simulink model "Cw2"  (R2016b)
settings: Solver=VariableStepDiscrete  StartTime=0.0  StopTime=2e-3  RelTol=1e-3
libraries: dspsrcs4 x4, dsparch4 x2, commutil2 x2, commchan3 x1, commseqgen3 x1
settings Model: Creator=Krzysztof  LastModifiedBy=Krzysztof

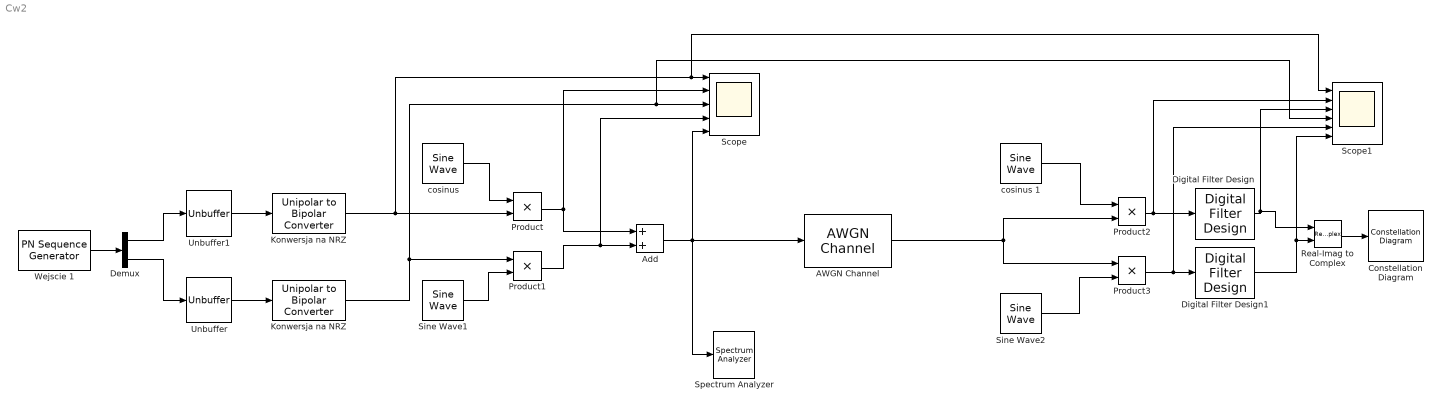
== system Cw2 ==
  AWGN Channel : commchan3/AWGN Channel  InputProcessing=Columns as channels (frame based)  seed=67  noiseMode="Signal to noise ratio  (Eb/No)"  EbNodB=20  EsNodB=10  SNRdB=30  bitsPerSym=2  Ps=1  Tsym=1/500e3  variance=1
  Add : Sum
  Constellation Diagram : ConstellationDiagram
  Demux : Demux  Outputs=2
  Digital Filter Design : dsparch4/Digital Filter Design  mwdsp_browser_bugfix_var=off
  Digital Filter Design1 : dsparch4/Digital Filter Design  mwdsp_browser_bugfix_var=off
  Konwersja na NRZ : commutil2/Unipolar to Bipolar Converter  M=2  polarity=Positive  dataType=Inherit via internal rule
  "Konwersja na NRZ " : commutil2/Unipolar to Bipolar Converter  M=2  polarity=Positive  dataType=Inherit via internal rule
  Product{,1..3} (4 alike) : Product
  Real-Imag to Complex : RealImagToComplex  SampleTime=1/400e6
  Scope : Scope  NumInputPorts=5
  Scope1 : Scope  NumInputPorts=6
  Sine Wave1 : dspsrcs4/Sine Wave  Amplitude=-1  Frequency=40e6  Phase=0  SampleMode=Discrete  OutComplex=Real  CompMethod=Trigonometric fcn  TableSize=Speed  SampleTime=1/400e6  SamplesPerFrame=1  ResetState=Restart at time zero  OutputFrames=off  dataType=double  wordLen=16  udDataType=sfix(16)  fracBitsMode=Best precision  numFracBits=15  OutDataTypeStr=double  LastOutDataTypeStr=double
  Sine Wave2 : dspsrcs4/Sine Wave  Amplitude=-1  Frequency=40e6  Phase=0  SampleMode=Discrete  OutComplex=Real  CompMethod=Trigonometric fcn  TableSize=Speed  SampleTime=1/400e6  SamplesPerFrame=1  ResetState=Restart at time zero  OutputFrames=off  dataType=double  wordLen=16  udDataType=sfix(16)  fracBitsMode=Best precision  numFracBits=15  OutDataTypeStr=double  LastOutDataTypeStr=double
  Spectrum Analyzer : SpectrumAnalyzer
  Unbuffer : Unbuffer  SampleBasedProcessing=Same as frame based
  Unbuffer1 : Unbuffer  SampleBasedProcessing=Same as frame based
  Wejscie 1 : commseqgen3/PN Sequence Generator  poly='z^7 + z^6 + 1'  ini_sta=[1 1 1 1 1 1 1]  outBitMaskSource=Dialog parameter  shift=0  outVarSiz=off  maxOutSizeMode=Dialog parameter  maxOutSize=[10 1]  Ts=1/1000e3  sampPerFrame=2  reset=off  bitPackedOutputs=off  outDataType=double  numPackedBits=8  bitPackDataSigned=off  bitPackedOutDType=double
  "cosinus " : dspsrcs4/Sine Wave  Amplitude=1  Frequency=40e6  Phase=pi/2  SampleMode=Discrete  OutComplex=Real  CompMethod=Trigonometric fcn  TableSize=Speed  SampleTime=1/400e6  SamplesPerFrame=1  ResetState=Restart at time zero  OutputFrames=off  dataType=double  wordLen=16  udDataType=sfix(16)  fracBitsMode=Best precision  numFracBits=15  OutDataTypeStr=double  LastOutDataTypeStr=double
  cosinus 1 : dspsrcs4/Sine Wave  Amplitude=1  Frequency=40e6  Phase=pi/2  SampleMode=Discrete  OutComplex=Real  CompMethod=Trigonometric fcn  TableSize=Speed  SampleTime=1/400e6  SamplesPerFrame=1  ResetState=Restart at time zero  OutputFrames=off  dataType=double  wordLen=16  udDataType=sfix(16)  fracBitsMode=Best precision  numFracBits=15  OutDataTypeStr=double  LastOutDataTypeStr=double
  wires:
  Unbuffer/1 -> "Konwersja na NRZ "/1
  Sine Wave1/1 -> Product1/2
  "Konwersja na NRZ "/1 -> Scope1/4, Scope/3, Product1/1
  Konwersja na NRZ/1 -> Scope1/1, Scope/1, Product/2
  "cosinus "/1 -> Product/1
  Product1/1 -> Scope/4, Add/2
  Product/1 -> Scope/2, Add/1
  AWGN Channel/1 -> Product3/1, Product2/2
  cosinus 1/1 -> Product2/1
  Sine Wave2/1 -> Product3/2
  Product3/1 -> Scope1/5, Digital Filter Design1/1
  Product2/1 -> Scope1/2, Digital Filter Design/1
  Digital Filter Design/1 -> Real-Imag to Complex/1, Scope1/3
  Digital Filter Design1/1 -> Real-Imag to Complex/2, Scope1/6
  Unbuffer1/1 -> Konwersja na NRZ/1
  Demux/1 -> Unbuffer1/1
  Demux/2 -> Unbuffer/1
  Wejscie 1/1 -> Demux/1
  Add/1 -> Spectrum Analyzer/1, AWGN Channel/1, Scope/5
  Real-Imag to Complex/1 -> Constellation Diagram/1
